simulink model "Heart"  (R2019a)
settings: Solver=VariableStepAuto  StartTime=0.0  StopTime=10.0  RelTol=1e-3
undefined symbols (not defined in the file): Q_gB, Q_gH, Q_gK, Q_gL, Q_gP, R_RBCU, V_gH
settings Model: Creator=jcp2  LastModifiedBy=jcp2

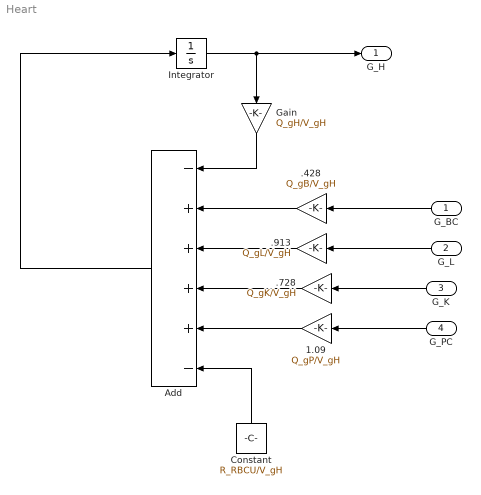
== system Heart ==
  G_BC : Inport
  G_L : Inport  Port=2
  G_K : Inport  Port=3
  G_PC : Inport  Port=4
  ".428 " : Gain  Gain=Q_gB/V_gH
  .728 : Gain  Gain=Q_gK/V_gH
  .913 : Gain  Gain=Q_gL/V_gH
  "1.09 " : Gain  Gain=Q_gP/V_gH
  Add : Sum  Inputs=-++++-
  Constant : Constant  Value=R_RBCU/V_gH
  Gain : Gain  Gain=Q_gH/V_gH
  Integrator : Integrator
  G_H : Outport
  wires:
  G_BC/1 -> ".428 "/1
  G_L/1 -> .913/1
  G_K/1 -> .728/1
  G_PC/1 -> "1.09 "/1
  Integrator/1 -> Gain/1, G_H/1
  Gain/1 -> Add/1
  Constant/1 -> Add/6
  "1.09 "/1 -> Add/5
  .728/1 -> Add/4
  .913/1 -> Add/3
  ".428 "/1 -> Add/2
  Add/1 -> Integrator/1
